simulink model "tankDrive"  (R2023b)
settings: Solver=FixedStepAuto  StartTime=0.0  StopTime=inf  RelTol=1e-3  EnableMultiTasking=on
libraries: vexarmcortexlib x4
settings Model: Creator=behja  LastModifiedBy=behja
settings DataIOCC: LimitDataPoints=on  SignalLoggingSaveFormat=ModelDataLogs  ReturnWorkspaceOutputs=off
settings OptimizationCC: ExpressionDepthLimit=2147483647  LifeSpan=Inf  MaxStackSize=64  EfficientTunableParamExpr=on
settings DebuggingCC: UnderspecifiedInitializationDetection=Classic  MergeDetectMultiDrivingBlocksExec=none  InheritedTsInSrcMsg=none  FcnCallInpInsideContextMsg=warning  StateNameClashWarn=warning  SFUnexpectedBacktrackingDiag=warning  SFNoUnconditionalDefaultTransitionDiag=warning  SFExecutionAtInitializationDiag=none  ArithmeticOperatorsInVariantConditions=warning
settings HardwareCC: ProdBitPerPointer=32  ProdBitPerSizeT=32  ProdBitPerPtrDiffT=32  ProdLargestAtomicInteger=Long  ProdLargestAtomicFloat=Double  ProdIntDivRoundTo=Undefined  ProdWordSize=32  ProdHWDeviceType=ARM Compatible->ARM Cortex
settings ModelReferenceCC: EnableRefExpFcnMdlSchedulingChecks=on  PropagateSignalLabelsOutOfModel=off
settings SFSimCC: MATLABDynamicMemAlloc=off  CustomCodeUndefinedFunction=UseInterfaceOnly
settings RTWCC: Description=Embedded Coder  SystemTargetFile=ert.tlc  HardwareBoard=ARM Cortex-based VEX Microcontroller  TemplateMakefile=ert_default_tmf  Toolchain=GNU Tools for VEX ARM Cortex
settings CodeAppCC: IgnoreCustomStorageClasses=off  CustomSymbolStrType=$N$R$M  StateflowObjectComments=on  InternalIdentifier=Classic
settings ERTTargetCC: CodeReplacementLibrary=GCC ARM Cortex-M3  MultiwordLength=2048  ConvertIfToSwitch=off  SuppressUnreachableDefaultCases=off

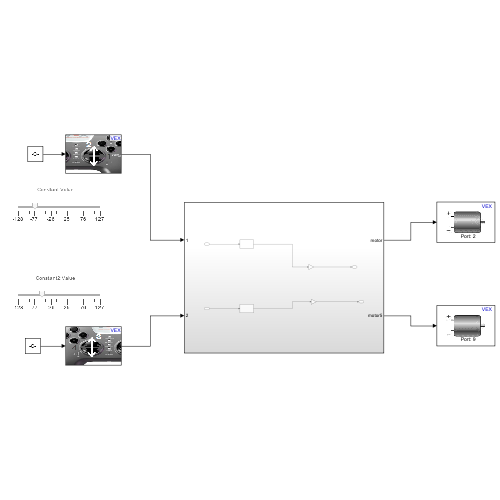
[thumbnail: Simulink's stored preview of the top-level diagram]
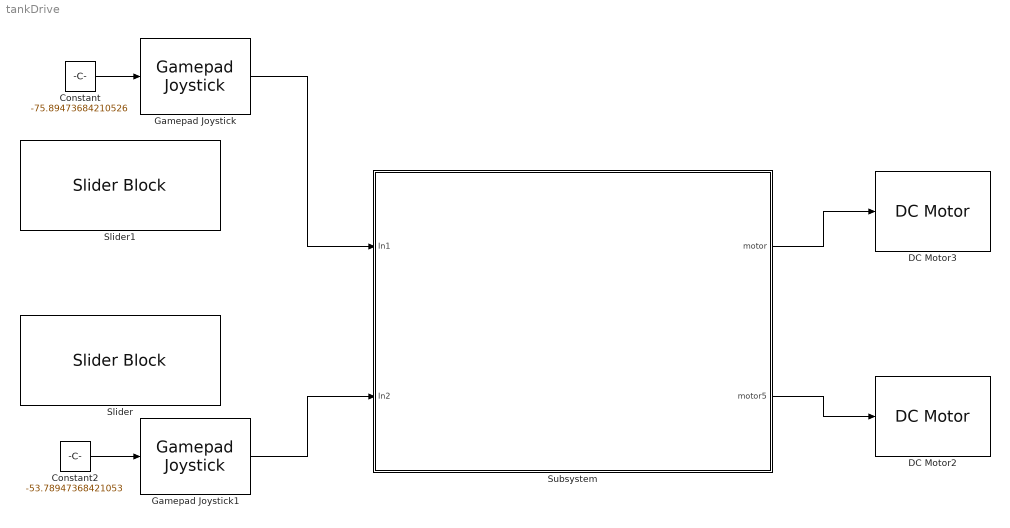
== system tankDrive ==
  Constant : Constant  Value=-75.89473684210526
  Constant2 : Constant  Value=-53.78947368421053
  DC Motor2 : vexarmcortexlib/Actuators/DC Motor  motor=9  scaleFactor=1/13.5  SimulationOut=off
  DC Motor3 : vexarmcortexlib/Actuators/DC Motor  motor=2  scaleFactor=1/13.5  SimulationOut=off
  Gamepad Joystick : vexarmcortexlib/Gamepad/Gamepad Joystick  joystick=1  chan=2  SimulationIn=on  SampleTime=0.02
  Gamepad Joystick1 : vexarmcortexlib/Gamepad/Gamepad Joystick  joystick=1  chan=3  SimulationIn=on  SampleTime=0.02
  Slider : SliderBlock  ScaleMin=-128  ScaleMax=127
  Slider1 : SliderBlock  ScaleMin=-128  ScaleMax=127
  Subsystem : Subsystem
  wires:
  Gamepad Joystick/1 -> Subsystem/1(In1)
  Constant/1 -> Gamepad Joystick/1
  Gamepad Joystick1/1 -> Subsystem/2(In2)
  Subsystem/2(motor5) -> DC Motor2/1
  Subsystem/1(motor) -> DC Motor3/1
  Constant2/1 -> Gamepad Joystick1/1

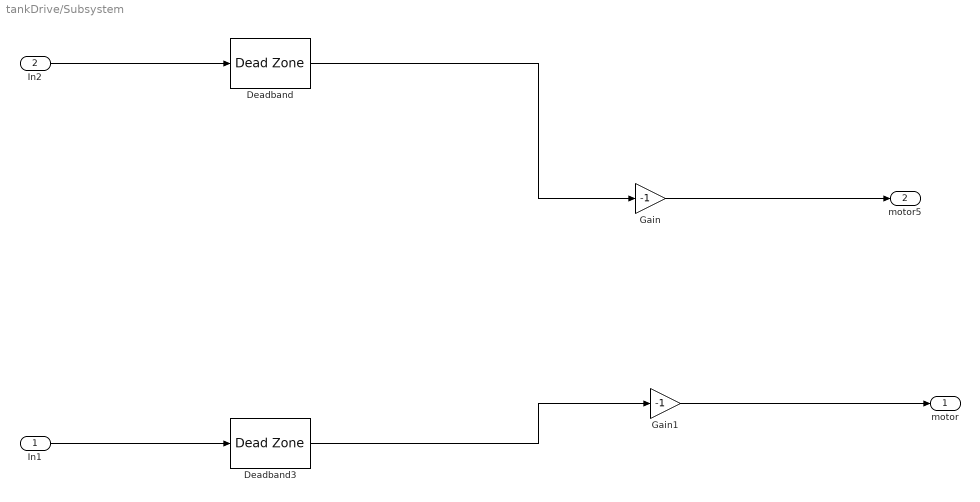
== system tankDrive/Subsystem ==
  In1 : Inport
  In2 : Inport  Port=2
  Deadband : DeadZone  LowerValue=-10  UpperValue=10
  Deadband3 : DeadZone  LowerValue=-10  UpperValue=10
  Gain : Gain  Gain=-1
  Gain1 : Gain  Gain=-1
  motor : Outport
  motor5 : Outport  Port=2
  wires:
  Gain1/1 -> motor/1
  Deadband3/1 -> Gain1/1
  Gain/1 -> motor5/1
  Deadband/1 -> Gain/1
  In1/1 -> Deadband3/1
  In2/1 -> Deadband/1
